simulink model "NGradosLibertadRetoSSControl"  (R2022a)
settings: Solver=VariableStepAuto  StartTime=0.0  StopTime=1000  RelTol=1e-3
undefined symbols (not defined in the file): b, G1, G2, G3, k, L1, L2, L3, m, mbkd_1, mbkd_2, mbkd_3, r_theta_1, r_theta_2, r_theta_3, z_0_1, z_0_2, z_0_3
settings Model: Creator=aafo_  LastModifiedBy=aafo_

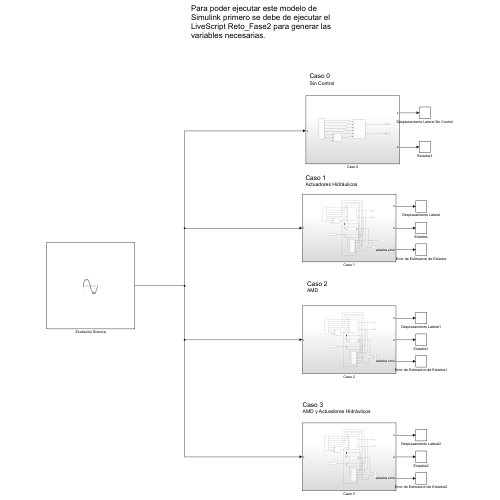
[thumbnail: Simulink's stored preview of the top-level diagram]
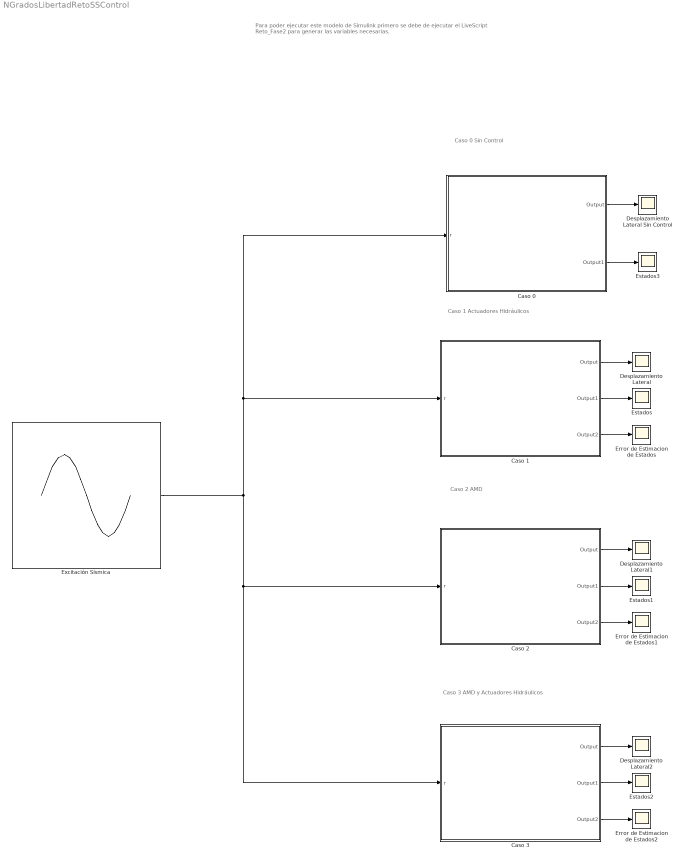
== system NGradosLibertadRetoSSControl ==
  note: Para poder ejecutar este modelo de Simulink primero se debe de ejecutar el LiveScript Reto_Fase2 para generar las variables necesarias.
  note: Caso 1
      | Actuadores Hidráulicos
  note: Caso 2
      | AMD
  note: Caso 3
      | AMD y Actuadores Hidráulicos
  note: Caso 0
      | Sin Control
  Caso 0 : Subsystem
  Caso 1 : Subsystem
  Caso 2 : Subsystem
  Caso 3 : Subsystem
  Desplazamiento Lateral : Scope
  Desplazamiento Lateral Sin Control : Scope
  Desplazamiento Lateral1 : Scope
  Desplazamiento Lateral2 : Scope
  Error de Estimacion de Estados : Scope
  Error de Estimacion de Estados1 : Scope
  Error de Estimacion de Estados2 : Scope
  Estados{,1..3} (4 alike) : Scope
  Excitación Sísmica : Sin  Frequency=14.6165  SampleTime=0
  wires:
  Caso 1/1(Output) -> Desplazamiento Lateral/1
  Caso 1/2(Output1) -> Estados/1
  Caso 1/3(Output2) -> Error de Estimacion de Estados/1
  Caso 2/1(Output) -> Desplazamiento Lateral1/1
  Caso 2/3(Output2) -> Error de Estimacion de Estados1/1
  Caso 2/2(Output1) -> Estados1/1
  Caso 3/2(Output1) -> Estados2/1
  Caso 3/3(Output2) -> Error de Estimacion de Estados2/1
  Caso 3/1(Output) -> Desplazamiento Lateral2/1
  Excitación Sísmica/1 -> Caso 0/1(r), Caso 1/1(r), Caso 3/1(r), Caso 2/1(r)
  Caso 0/2(Output1) -> Estados3/1
  Caso 0/1(Output) -> Desplazamiento Lateral Sin Control/1

== system NGradosLibertadRetoSSControl/Caso 0 ==
  note: Perturbación
  r : Inport
  Parámetros del Sistema : Subsystem
  Perturbacion Matricial : MATLAB Function  TreatAsAtomicUnit=on
  Sistema En Espacio de Estados : Subsystem
  Output : Outport
  Output1 : Outport  Port=2
  wires:
  Perturbacion Matricial/1(out) -> Sistema En Espacio de Estados/6(Perturbación)  "rm"
  Sistema En Espacio de Estados/2(Output6) -> Output1/1  "z"
  Sistema En Espacio de Estados/1(Output5) -> Output/1  "x"
  Parámetros del Sistema/5(Bu) -> Sistema En Espacio de Estados/5(Input4)
  Parámetros del Sistema/3(C) -> Sistema En Espacio de Estados/3(Input2)
  Parámetros del Sistema/1(A) -> Sistema En Espacio de Estados/1(Input)
  Parámetros del Sistema/2(Br) -> Sistema En Espacio de Estados/2(Input1)
  Parámetros del Sistema/7(Output1) -> Perturbacion Matricial/2(m)
  Parámetros del Sistema/4(D) -> Sistema En Espacio de Estados/4(Input3)
  Parámetros del Sistema/6(Output) -> Perturbacion Matricial/1(mbkd)
  r/1 -> Perturbacion Matricial/3(r)

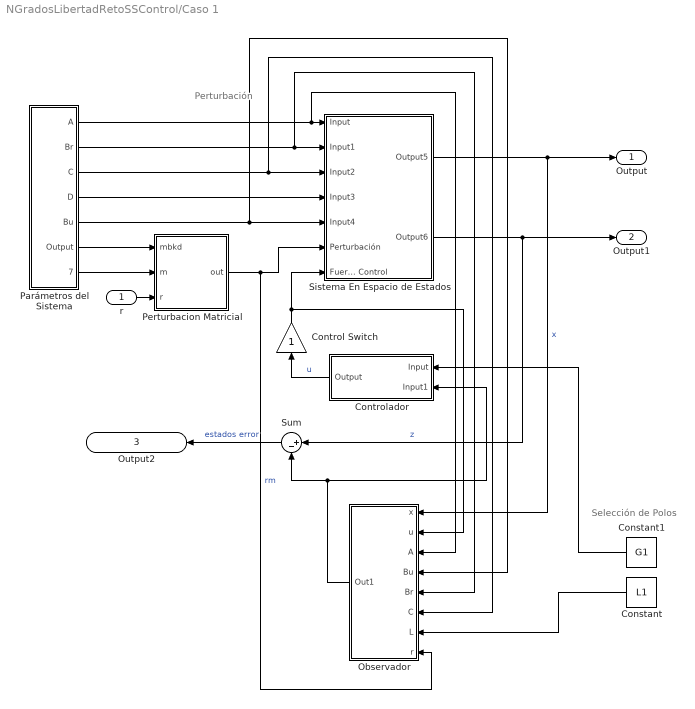
== system NGradosLibertadRetoSSControl/Caso 1 ==
  note: Selección de Polos
  note: Perturbación
  r : Inport
  Constant : Constant  Value=L1
  Constant1 : Constant  Value=G1
  Control Switch : Gain
  Controlador : Subsystem
  Observador : Subsystem
  Parámetros del Sistema : Subsystem
  Perturbacion Matricial : MATLAB Function  TreatAsAtomicUnit=on
  Sistema En Espacio de Estados : Subsystem
  Sum : Sum  Inputs=|+-
  Output : Outport
  Output1 : Outport  Port=2
  Output2 : Outport  Port=3
  wires:
  Observador/1(Out1) -> Controlador/2(Input1), Sum/2
  Sum/1 -> Output2/1  "estados error"
  Perturbacion Matricial/1(out) -> Sistema En Espacio de Estados/6(Perturbación), Observador/8(r)  "rm"
  Sistema En Espacio de Estados/2(Output6) -> Output1/1, Sum/1  "z"
  Sistema En Espacio de Estados/1(Output5) -> Output/1, Observador/1(x)  "x"
  Controlador/1(Output) -> Control Switch/1  "u"
  Parámetros del Sistema/5(Bu) -> Sistema En Espacio de Estados/5(Input4), Observador/4(Bu)
  Parámetros del Sistema/3(C) -> Sistema En Espacio de Estados/3(Input2), Observador/6(C)
  Constant1/1 -> Controlador/1(Input)
  Parámetros del Sistema/1(A) -> Observador/3(A), Sistema En Espacio de Estados/1(Input)
  Parámetros del Sistema/2(Br) -> Sistema En Espacio de Estados/2(Input1), Observador/5(Br)
  Constant/1 -> Observador/7(L)
  Parámetros del Sistema/7(Output1) -> Perturbacion Matricial/2(m)
  Parámetros del Sistema/4(D) -> Sistema En Espacio de Estados/4(Input3)
  Parámetros del Sistema/6(Output) -> Perturbacion Matricial/1(mbkd)
  r/1 -> Perturbacion Matricial/3(r)
  Control Switch/1 -> Sistema En Espacio de Estados/7(Fuerza De Control), Observador/2(u)

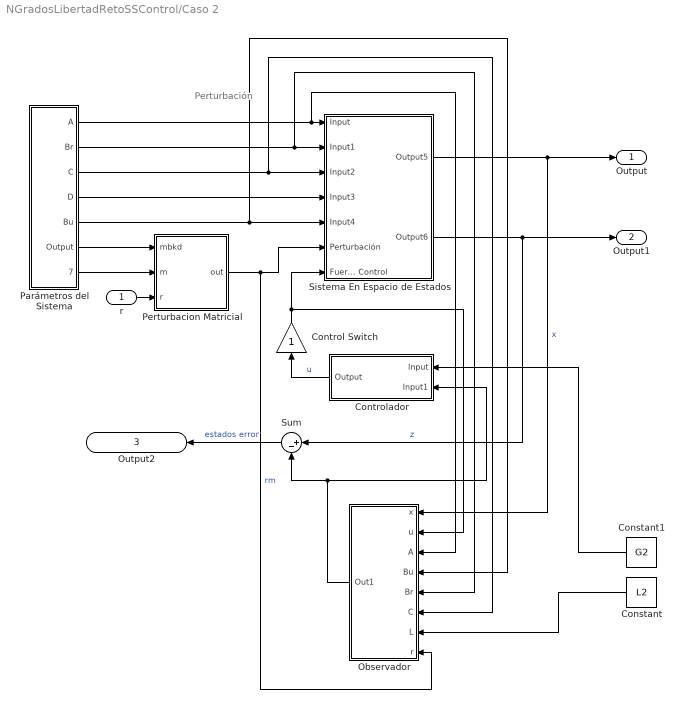
== system NGradosLibertadRetoSSControl/Caso 2 ==
  note: Perturbación
  r : Inport
  Constant : Constant  Value=L2
  Constant1 : Constant  Value=G2
  Control Switch : Gain
  Controlador : Subsystem
  Observador : Subsystem
  Parámetros del Sistema : Subsystem
  Perturbacion Matricial : MATLAB Function  TreatAsAtomicUnit=on
  Sistema En Espacio de Estados : Subsystem
  Sum : Sum  Inputs=|+-
  Output : Outport
  Output1 : Outport  Port=2
  Output2 : Outport  Port=3
  wires:
  Observador/1(Out1) -> Controlador/2(Input1), Sum/2
  Sum/1 -> Output2/1  "estados error"
  Perturbacion Matricial/1(out) -> Sistema En Espacio de Estados/6(Perturbación), Observador/8(r)  "rm"
  Sistema En Espacio de Estados/2(Output6) -> Output1/1, Sum/1  "z"
  Sistema En Espacio de Estados/1(Output5) -> Output/1, Observador/1(x)  "x"
  Controlador/1(Output) -> Control Switch/1  "u"
  Parámetros del Sistema/5(Bu) -> Sistema En Espacio de Estados/5(Input4), Observador/4(Bu)
  Parámetros del Sistema/3(C) -> Sistema En Espacio de Estados/3(Input2), Observador/6(C)
  Constant1/1 -> Controlador/1(Input)
  Parámetros del Sistema/1(A) -> Observador/3(A), Sistema En Espacio de Estados/1(Input)
  Parámetros del Sistema/2(Br) -> Sistema En Espacio de Estados/2(Input1), Observador/5(Br)
  Constant/1 -> Observador/7(L)
  Parámetros del Sistema/7(Output1) -> Perturbacion Matricial/2(m)
  Parámetros del Sistema/4(D) -> Sistema En Espacio de Estados/4(Input3)
  Parámetros del Sistema/6(Output) -> Perturbacion Matricial/1(mbkd)
  r/1 -> Perturbacion Matricial/3(r)
  Control Switch/1 -> Sistema En Espacio de Estados/7(Fuerza De Control), Observador/2(u)

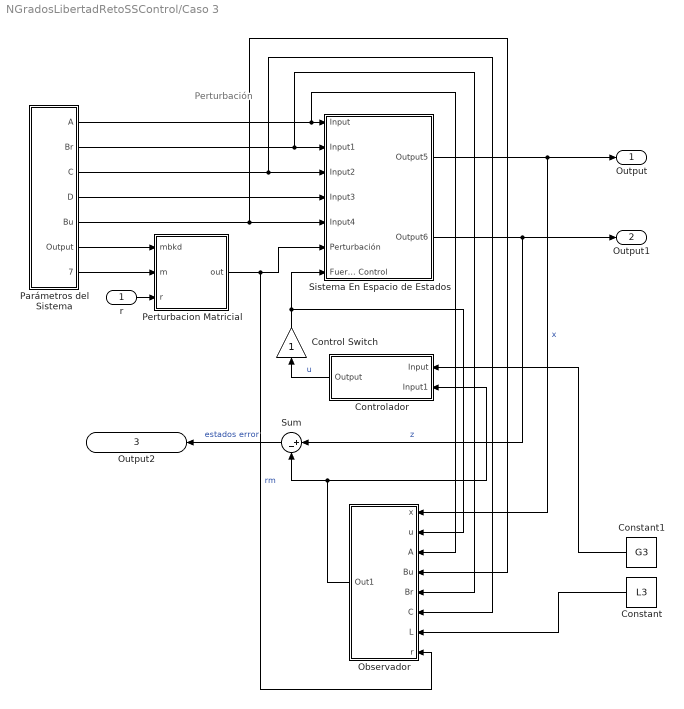
== system NGradosLibertadRetoSSControl/Caso 3 ==
  note: Perturbación
  r : Inport
  Constant : Constant  Value=L3
  Constant1 : Constant  Value=G3
  Control Switch : Gain
  Controlador : Subsystem
  Observador : Subsystem
  Parámetros del Sistema : Subsystem
  Perturbacion Matricial : MATLAB Function  TreatAsAtomicUnit=on
  Sistema En Espacio de Estados : Subsystem
  Sum : Sum  Inputs=|+-
  Output : Outport
  Output1 : Outport  Port=2
  Output2 : Outport  Port=3
  wires:
  Observador/1(Out1) -> Controlador/2(Input1), Sum/2
  Sum/1 -> Output2/1  "estados error"
  Perturbacion Matricial/1(out) -> Sistema En Espacio de Estados/6(Perturbación), Observador/8(r)  "rm"
  Sistema En Espacio de Estados/2(Output6) -> Output1/1, Sum/1  "z"
  Sistema En Espacio de Estados/1(Output5) -> Output/1, Observador/1(x)  "x"
  Controlador/1(Output) -> Control Switch/1  "u"
  Parámetros del Sistema/5(Bu) -> Sistema En Espacio de Estados/5(Input4), Observador/4(Bu)
  Parámetros del Sistema/3(C) -> Sistema En Espacio de Estados/3(Input2), Observador/6(C)
  Constant1/1 -> Controlador/1(Input)
  Parámetros del Sistema/1(A) -> Observador/3(A), Sistema En Espacio de Estados/1(Input)
  Parámetros del Sistema/2(Br) -> Sistema En Espacio de Estados/2(Input1), Observador/5(Br)
  Constant/1 -> Observador/7(L)
  Parámetros del Sistema/7(Output1) -> Perturbacion Matricial/2(m)
  Parámetros del Sistema/4(D) -> Sistema En Espacio de Estados/4(Input3)
  Parámetros del Sistema/6(Output) -> Perturbacion Matricial/1(mbkd)
  r/1 -> Perturbacion Matricial/3(r)
  Control Switch/1 -> Sistema En Espacio de Estados/7(Fuerza De Control), Observador/2(u)

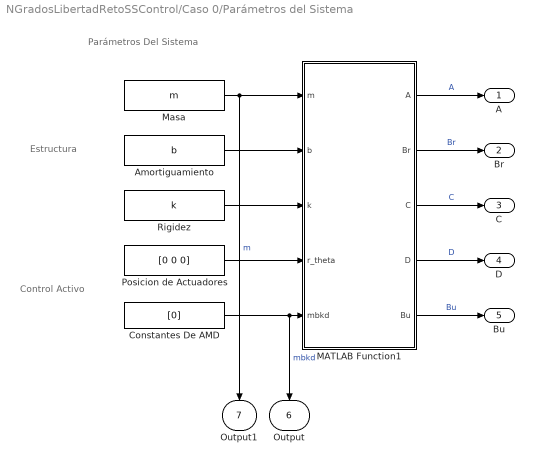
== system NGradosLibertadRetoSSControl/Caso 0/Parámetros del Sistema ==
  note: Control Activo
  note: Estructura
  note: Parámetros Del Sistema
  Amortiguamiento : Constant  Value=b
  Constantes De AMD : Constant  Value=[0]
  MATLAB Function1 : MATLAB Function  TreatAsAtomicUnit=on
  Masa : Constant  Value=m
  Posicion de Actuadores : Constant  Value=[0 0 0]
  Rigidez : Constant  Value=k
  A : Outport
  Br : Outport  Port=2
  C : Outport  Port=3
  D : Outport  Port=4
  Bu : Outport  Port=5
  Output : Outport  Port=6
  Output1 : Outport  Port=7
  wires:
  Masa/1 -> MATLAB Function1/1(m), Output1/1  "m"
  Constantes De AMD/1 -> MATLAB Function1/5(mbkd), Output/1  "mbkd"
  MATLAB Function1/1(A) -> A/1  "A"
  Amortiguamiento/1 -> MATLAB Function1/2(b)
  Rigidez/1 -> MATLAB Function1/3(k)
  Posicion de Actuadores/1 -> MATLAB Function1/4(r_theta)
  MATLAB Function1/2(Br) -> Br/1  "Br"
  MATLAB Function1/3(C) -> C/1  "C"
  MATLAB Function1/4(D) -> D/1  "D"
  MATLAB Function1/5(Bu) -> Bu/1  "Bu"

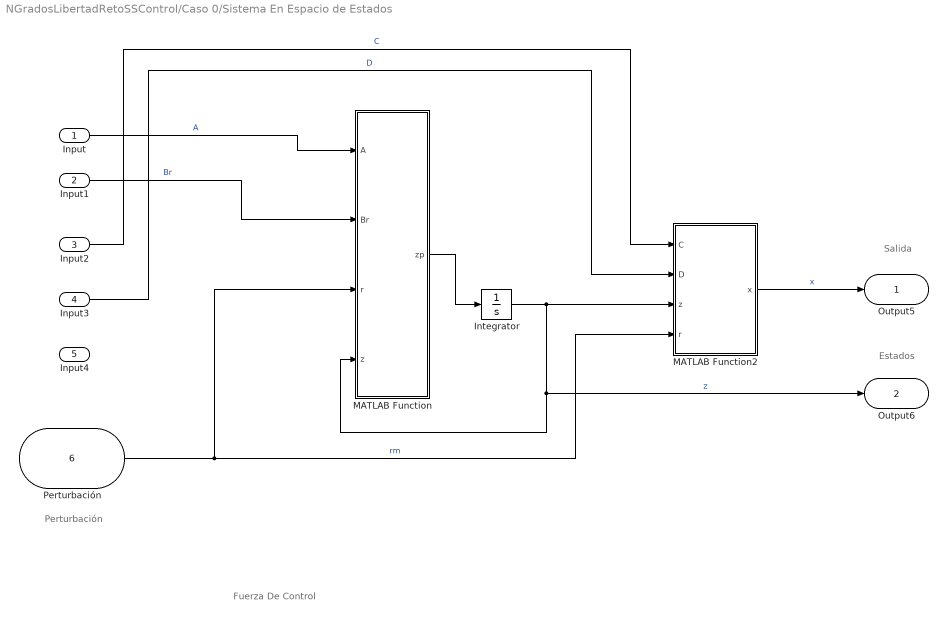
== system NGradosLibertadRetoSSControl/Caso 0/Sistema En Espacio de Estados ==
  note: Estados
  note: Fuerza De Control
  note: Perturbación
  note: Salida
  Input : Inport
  Input1 : Inport  Port=2
  Input2 : Inport  Port=3
  Input3 : Inport  Port=4
  Input4 : Inport  Port=5
  Perturbación : Inport  Port=6
  Integrator : Integrator  InitialCondition=z_0_1
  MATLAB Function : MATLAB Function  TreatAsAtomicUnit=on
  MATLAB Function2 : MATLAB Function  TreatAsAtomicUnit=on
  Output5 : Outport
  Output6 : Outport  Port=2
  wires:
  Integrator/1 -> MATLAB Function/4(z), Output6/1, MATLAB Function2/3(z)  "z"
  Input3/1 -> MATLAB Function2/2(D)  "D"
  Input1/1 -> MATLAB Function/2(Br)  "Br"
  Input/1 -> MATLAB Function/1(A)  "A"
  MATLAB Function/1(zp) -> Integrator/1
  Input2/1 -> MATLAB Function2/1(C)  "C"
  Perturbación/1 -> MATLAB Function2/4(r), MATLAB Function/3(r)  "rm"
  MATLAB Function2/1(x) -> Output5/1  "x"

== system NGradosLibertadRetoSSControl/Caso 1/Controlador ==
  Input : Inport
  Input1 : Inport  Port=2
  Gain : Gain  Gain=-1
  Matrix Multiply : Product  Multiplication=Matrix(*)
  Output : Outport
  wires:
  Input/1 -> Matrix Multiply/1  "G"
  Matrix Multiply/1 -> Gain/1
  Input1/1 -> Matrix Multiply/2  "z"
  Gain/1 -> Output/1  "u"

== system NGradosLibertadRetoSSControl/Caso 1/Observador ==
  x : Inport
  u : Inport  Port=2
  A : Inport  Port=3
  Bu : Inport  Port=4
  Br : Inport  Port=5
  C : Inport  Port=6
  L : Inport  Port=7
  r : Inport  Port=8
  Integrator : Integrator  InitialCondition=z_0_1
  MATLAB Function : MATLAB Function  TreatAsAtomicUnit=on
  Out1 : Outport
  wires:
  Bu/1 -> MATLAB Function/2(Bu)
  MATLAB Function/1(zp_est) -> Integrator/1  "zpest"
  Integrator/1 -> MATLAB Function/9(zest), Out1/1  "zest"
  L/1 -> MATLAB Function/5(L)
  A/1 -> MATLAB Function/1(A)
  Br/1 -> MATLAB Function/3(Br)
  C/1 -> MATLAB Function/4(C)
  r/1 -> MATLAB Function/7(r)
  u/1 -> MATLAB Function/6(u)
  x/1 -> MATLAB Function/8(x)

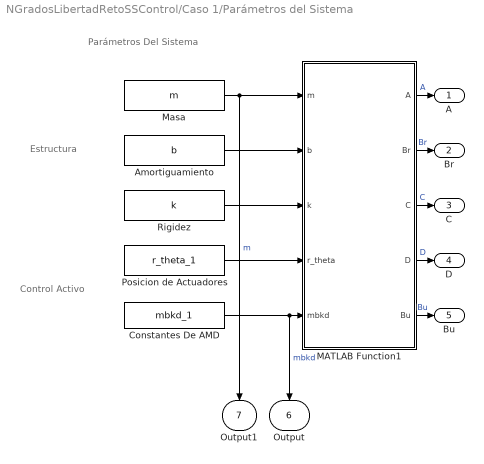
== system NGradosLibertadRetoSSControl/Caso 1/Parámetros del Sistema ==
  note: Control Activo
  note: Estructura
  note: Parámetros Del Sistema
  Amortiguamiento : Constant  Value=b
  Constantes De AMD : Constant  Value=mbkd_1
  MATLAB Function1 : MATLAB Function  TreatAsAtomicUnit=on
  Masa : Constant  Value=m
  Posicion de Actuadores : Constant  Value=r_theta_1
  Rigidez : Constant  Value=k
  A : Outport
  Br : Outport  Port=2
  C : Outport  Port=3
  D : Outport  Port=4
  Bu : Outport  Port=5
  Output : Outport  Port=6
  Output1 : Outport  Port=7
  wires:
  Masa/1 -> MATLAB Function1/1(m), Output1/1  "m"
  Constantes De AMD/1 -> MATLAB Function1/5(mbkd), Output/1  "mbkd"
  MATLAB Function1/1(A) -> A/1  "A"
  Amortiguamiento/1 -> MATLAB Function1/2(b)
  Rigidez/1 -> MATLAB Function1/3(k)
  Posicion de Actuadores/1 -> MATLAB Function1/4(r_theta)
  MATLAB Function1/2(Br) -> Br/1  "Br"
  MATLAB Function1/3(C) -> C/1  "C"
  MATLAB Function1/4(D) -> D/1  "D"
  MATLAB Function1/5(Bu) -> Bu/1  "Bu"

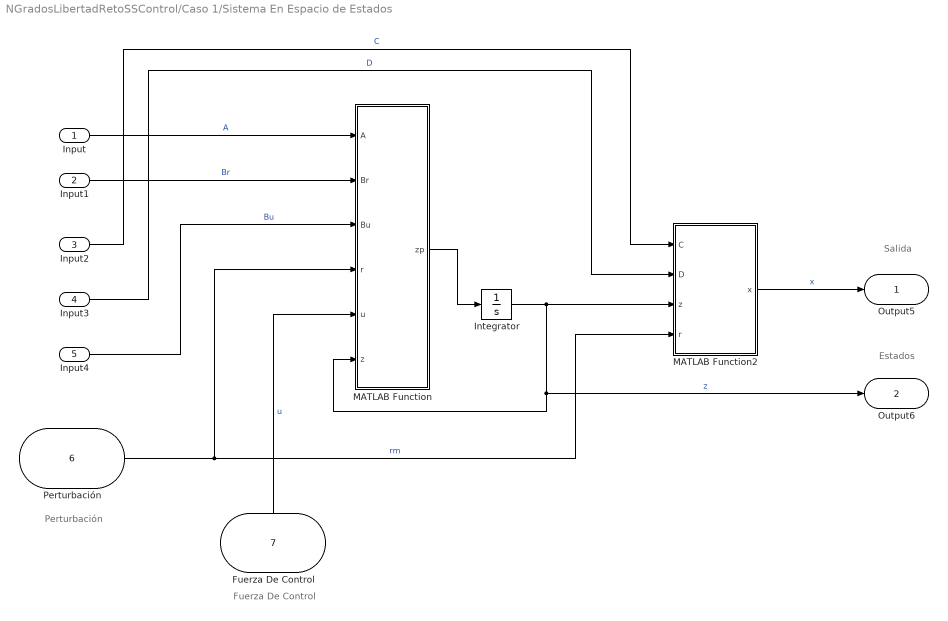
== system NGradosLibertadRetoSSControl/Caso 1/Sistema En Espacio de Estados ==
  note: Estados
  note: Fuerza De Control
  note: Perturbación
  note: Salida
  Input : Inport
  Input1 : Inport  Port=2
  Input2 : Inport  Port=3
  Input3 : Inport  Port=4
  Input4 : Inport  Port=5
  Perturbación : Inport  Port=6
  Fuerza De Control : Inport  Port=7
  Integrator : Integrator  InitialCondition=z_0_1
  MATLAB Function : MATLAB Function  TreatAsAtomicUnit=on
  MATLAB Function2 : MATLAB Function  TreatAsAtomicUnit=on
  Output5 : Outport
  Output6 : Outport  Port=2
  wires:
  Integrator/1 -> MATLAB Function/6(z), Output6/1, MATLAB Function2/3(z)  "z"
  Input3/1 -> MATLAB Function2/2(D)  "D"
  Input1/1 -> MATLAB Function/2(Br)  "Br"
  Input/1 -> MATLAB Function/1(A)  "A"
  MATLAB Function/1(zp) -> Integrator/1
  Input2/1 -> MATLAB Function2/1(C)  "C"
  Perturbación/1 -> MATLAB Function2/4(r), MATLAB Function/4(r)  "rm"
  MATLAB Function2/1(x) -> Output5/1  "x"
  Input4/1 -> MATLAB Function/3(Bu)  "Bu"
  Fuerza De Control/1 -> MATLAB Function/5(u)  "u"

== system NGradosLibertadRetoSSControl/Caso 2/Controlador ==
  Input : Inport
  Input1 : Inport  Port=2
  Gain : Gain  Gain=-1
  Matrix Multiply : Product  Multiplication=Matrix(*)
  Output : Outport
  wires:
  Input/1 -> Matrix Multiply/1  "G"
  Matrix Multiply/1 -> Gain/1
  Input1/1 -> Matrix Multiply/2  "z"
  Gain/1 -> Output/1  "u"

== system NGradosLibertadRetoSSControl/Caso 2/Observador ==
  x : Inport
  u : Inport  Port=2
  A : Inport  Port=3
  Bu : Inport  Port=4
  Br : Inport  Port=5
  C : Inport  Port=6
  L : Inport  Port=7
  r : Inport  Port=8
  Integrator : Integrator  InitialCondition=z_0_2
  MATLAB Function : MATLAB Function  TreatAsAtomicUnit=on
  Out1 : Outport
  wires:
  Bu/1 -> MATLAB Function/2(Bu)
  MATLAB Function/1(zp_est) -> Integrator/1  "zpest"
  Integrator/1 -> MATLAB Function/9(zest), Out1/1  "zest"
  L/1 -> MATLAB Function/5(L)
  A/1 -> MATLAB Function/1(A)
  Br/1 -> MATLAB Function/3(Br)
  C/1 -> MATLAB Function/4(C)
  r/1 -> MATLAB Function/7(r)
  u/1 -> MATLAB Function/6(u)
  x/1 -> MATLAB Function/8(x)

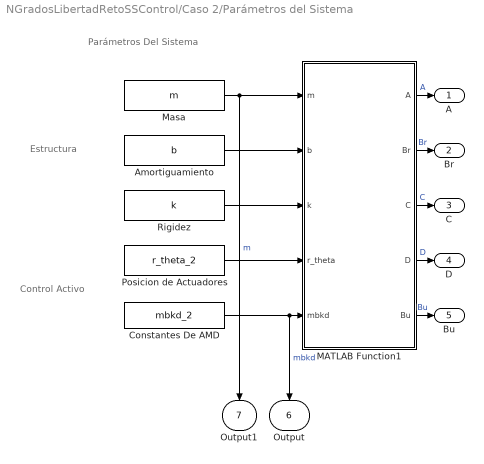
== system NGradosLibertadRetoSSControl/Caso 2/Parámetros del Sistema ==
  note: Control Activo
  note: Estructura
  note: Parámetros Del Sistema
  Amortiguamiento : Constant  Value=b
  Constantes De AMD : Constant  Value=mbkd_2
  MATLAB Function1 : MATLAB Function  TreatAsAtomicUnit=on
  Masa : Constant  Value=m
  Posicion de Actuadores : Constant  Value=r_theta_2
  Rigidez : Constant  Value=k
  A : Outport
  Br : Outport  Port=2
  C : Outport  Port=3
  D : Outport  Port=4
  Bu : Outport  Port=5
  Output : Outport  Port=6
  Output1 : Outport  Port=7
  wires:
  Masa/1 -> MATLAB Function1/1(m), Output1/1  "m"
  Constantes De AMD/1 -> MATLAB Function1/5(mbkd), Output/1  "mbkd"
  MATLAB Function1/1(A) -> A/1  "A"
  Amortiguamiento/1 -> MATLAB Function1/2(b)
  Rigidez/1 -> MATLAB Function1/3(k)
  Posicion de Actuadores/1 -> MATLAB Function1/4(r_theta)
  MATLAB Function1/2(Br) -> Br/1  "Br"
  MATLAB Function1/3(C) -> C/1  "C"
  MATLAB Function1/4(D) -> D/1  "D"
  MATLAB Function1/5(Bu) -> Bu/1  "Bu"

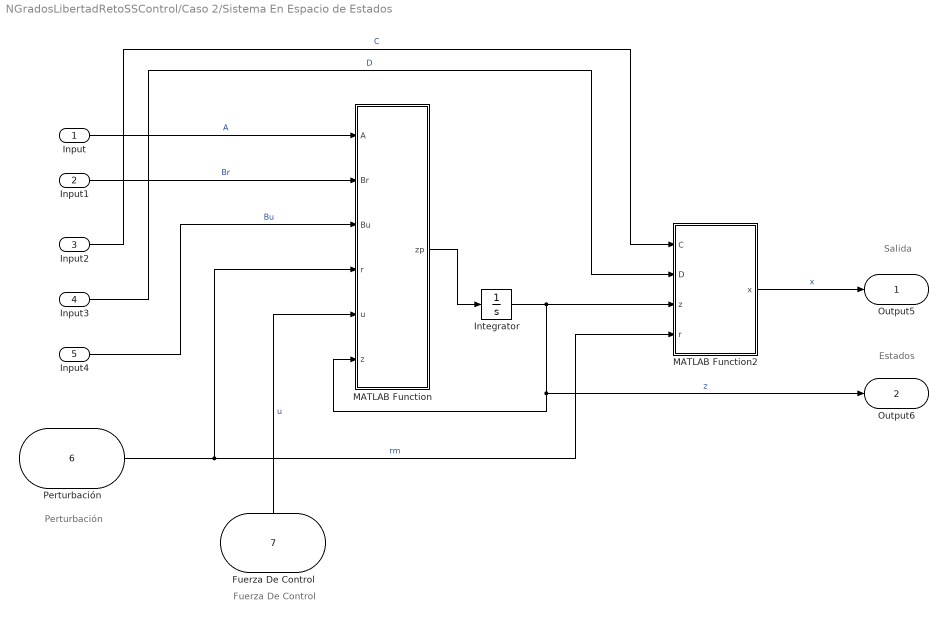
== system NGradosLibertadRetoSSControl/Caso 2/Sistema En Espacio de Estados ==
  note: Estados
  note: Fuerza De Control
  note: Perturbación
  note: Salida
  Input : Inport
  Input1 : Inport  Port=2
  Input2 : Inport  Port=3
  Input3 : Inport  Port=4
  Input4 : Inport  Port=5
  Perturbación : Inport  Port=6
  Fuerza De Control : Inport  Port=7
  Integrator : Integrator  InitialCondition=z_0_2
  MATLAB Function : MATLAB Function  TreatAsAtomicUnit=on
  MATLAB Function2 : MATLAB Function  TreatAsAtomicUnit=on
  Output5 : Outport
  Output6 : Outport  Port=2
  wires:
  Integrator/1 -> MATLAB Function/6(z), Output6/1, MATLAB Function2/3(z)  "z"
  Input3/1 -> MATLAB Function2/2(D)  "D"
  Input1/1 -> MATLAB Function/2(Br)  "Br"
  Input/1 -> MATLAB Function/1(A)  "A"
  MATLAB Function/1(zp) -> Integrator/1
  Input2/1 -> MATLAB Function2/1(C)  "C"
  Perturbación/1 -> MATLAB Function2/4(r), MATLAB Function/4(r)  "rm"
  MATLAB Function2/1(x) -> Output5/1  "x"
  Input4/1 -> MATLAB Function/3(Bu)  "Bu"
  Fuerza De Control/1 -> MATLAB Function/5(u)  "u"

== system NGradosLibertadRetoSSControl/Caso 3/Controlador ==
  Input : Inport
  Input1 : Inport  Port=2
  Gain : Gain  Gain=-1
  Matrix Multiply : Product  Multiplication=Matrix(*)
  Output : Outport
  wires:
  Input/1 -> Matrix Multiply/1  "G"
  Matrix Multiply/1 -> Gain/1
  Input1/1 -> Matrix Multiply/2  "z"
  Gain/1 -> Output/1  "u"

== system NGradosLibertadRetoSSControl/Caso 3/Observador ==
  x : Inport
  u : Inport  Port=2
  A : Inport  Port=3
  Bu : Inport  Port=4
  Br : Inport  Port=5
  C : Inport  Port=6
  L : Inport  Port=7
  r : Inport  Port=8
  Integrator : Integrator  InitialCondition=z_0_3
  MATLAB Function : MATLAB Function  TreatAsAtomicUnit=on
  Out1 : Outport
  wires:
  Bu/1 -> MATLAB Function/2(Bu)
  MATLAB Function/1(zp_est) -> Integrator/1  "zpest"
  Integrator/1 -> MATLAB Function/9(zest), Out1/1  "zest"
  L/1 -> MATLAB Function/5(L)
  A/1 -> MATLAB Function/1(A)
  Br/1 -> MATLAB Function/3(Br)
  C/1 -> MATLAB Function/4(C)
  r/1 -> MATLAB Function/7(r)
  u/1 -> MATLAB Function/6(u)
  x/1 -> MATLAB Function/8(x)

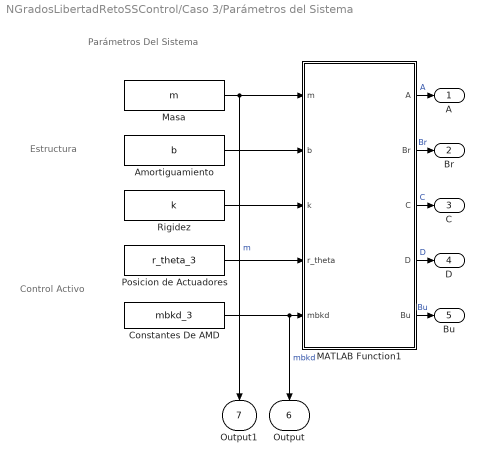
== system NGradosLibertadRetoSSControl/Caso 3/Parámetros del Sistema ==
  note: Control Activo
  note: Estructura
  note: Parámetros Del Sistema
  Amortiguamiento : Constant  Value=b
  Constantes De AMD : Constant  Value=mbkd_3
  MATLAB Function1 : MATLAB Function  TreatAsAtomicUnit=on
  Masa : Constant  Value=m
  Posicion de Actuadores : Constant  Value=r_theta_3
  Rigidez : Constant  Value=k
  A : Outport
  Br : Outport  Port=2
  C : Outport  Port=3
  D : Outport  Port=4
  Bu : Outport  Port=5
  Output : Outport  Port=6
  Output1 : Outport  Port=7
  wires:
  Masa/1 -> MATLAB Function1/1(m), Output1/1  "m"
  Constantes De AMD/1 -> MATLAB Function1/5(mbkd), Output/1  "mbkd"
  MATLAB Function1/1(A) -> A/1  "A"
  Amortiguamiento/1 -> MATLAB Function1/2(b)
  Rigidez/1 -> MATLAB Function1/3(k)
  Posicion de Actuadores/1 -> MATLAB Function1/4(r_theta)
  MATLAB Function1/2(Br) -> Br/1  "Br"
  MATLAB Function1/3(C) -> C/1  "C"
  MATLAB Function1/4(D) -> D/1  "D"
  MATLAB Function1/5(Bu) -> Bu/1  "Bu"

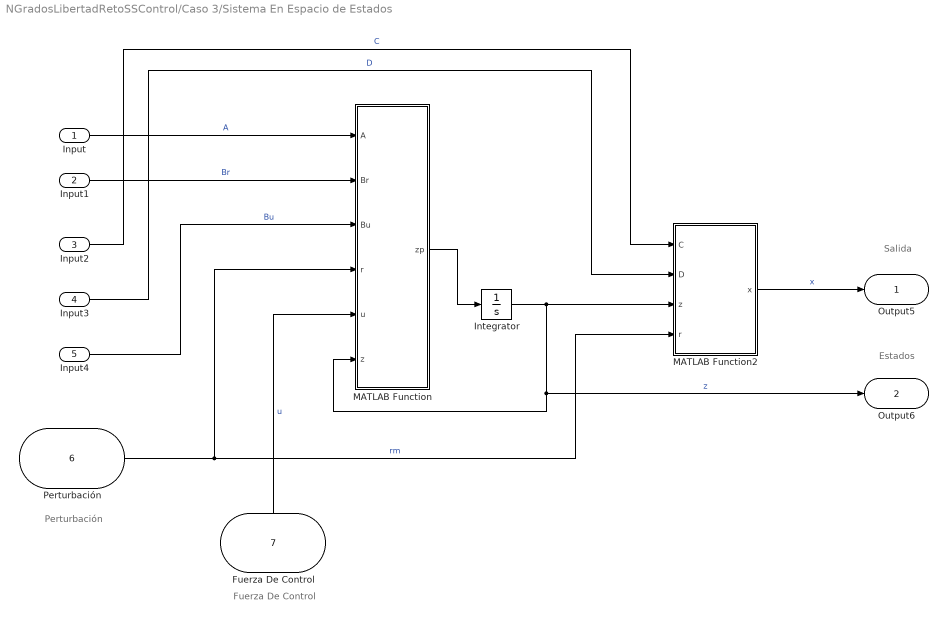
== system NGradosLibertadRetoSSControl/Caso 3/Sistema En Espacio de Estados ==
  note: Estados
  note: Fuerza De Control
  note: Perturbación
  note: Salida
  Input : Inport
  Input1 : Inport  Port=2
  Input2 : Inport  Port=3
  Input3 : Inport  Port=4
  Input4 : Inport  Port=5
  Perturbación : Inport  Port=6
  Fuerza De Control : Inport  Port=7
  Integrator : Integrator  InitialCondition=z_0_3
  MATLAB Function : MATLAB Function  TreatAsAtomicUnit=on
  MATLAB Function2 : MATLAB Function  TreatAsAtomicUnit=on
  Output5 : Outport
  Output6 : Outport  Port=2
  wires:
  Integrator/1 -> MATLAB Function/6(z), Output6/1, MATLAB Function2/3(z)  "z"
  Input3/1 -> MATLAB Function2/2(D)  "D"
  Input1/1 -> MATLAB Function/2(Br)  "Br"
  Input/1 -> MATLAB Function/1(A)  "A"
  MATLAB Function/1(zp) -> Integrator/1
  Input2/1 -> MATLAB Function2/1(C)  "C"
  Perturbación/1 -> MATLAB Function2/4(r), MATLAB Function/4(r)  "rm"
  MATLAB Function2/1(x) -> Output5/1  "x"
  Input4/1 -> MATLAB Function/3(Bu)  "Bu"
  Fuerza De Control/1 -> MATLAB Function/5(u)  "u"

== matlab function NGradosLibertadRetoSSControl/Caso 2/Perturbacion Matricial ==
  data: mbkd input; m input; r input; out output
function out = rMatrix(mbkd, m,r)
n = length(m);
if length(mbkd) == 3

    out = r.*ones(n+1,1);
else
    out = r.*ones(n,1);
end

== matlab function NGradosLibertadRetoSSControl/Caso 2/Sistema En Espacio de Estados/MATLAB Function ==
  data: A input; Br input; Bu input; r input; u input; z input; zp output
function zp = StatesModel(A , Br, Bu, r, u, z)

zp = A*z+Br*r+ Bu*u;

== matlab function NGradosLibertadRetoSSControl/Caso 2/Sistema En Espacio de Estados/MATLAB Function2 ==
  data: C input; D input; z input; x output; r input
function x = StatesToX(C, D, z, r)

x = C*z+ D*r;

== matlab function NGradosLibertadRetoSSControl/Caso 3/Observador/MATLAB Function ==
  data: A input; Bu input; Br input; C input; L input; u input; zp_est output; r input; x input; zest input
function zp_est = fcn(A, Bu, Br, C, L, u, r, x, zest)

xerr = x-C*zest;
zp_est = A*zest + Bu*u + Br*r + L*xerr;

== matlab function NGradosLibertadRetoSSControl/Caso 3/Parámetros del Sistema/MATLAB Function1 ==
  data: m input; A output; b input; k input; r_theta input; Br output; C output; D output; Bu output; mbkd input
function [A, Br, C, D, Bu] = StatesModelMatrix(m, b, k, r_theta, mbkd)
if length(mbkd) == 3
%% AMD
    md = mbkd(1); bd = mbkd(2); kd = mbkd(3);

    M = MM_AMD(MM(m),md);
    
    B_ = BK_AMD(BK(b),bd);
    
    K = BK_AMD(BK(k),kd);
    
    delta = -1*[m' md]';
    
    nn = size(M, 1);
    
    gamma = gamma_AMD(gamma_bar(length(m))*MM(r_theta));
    
    A = [zeros(nn) eye(nn); -inv(M)*K -inv(M)*B_];
    
    Br = [zeros(nn);MM(inv(M)*delta)];
    
    Bu = [zeros(nn); inv(M)*gamma];
    
    C = [eye(nn) zeros(nn)];
    
    D = zeros(nn);

%% Sin AMD
else

    M = MM(m);
    
    B_ = BK(b);
    
    K = BK(k);
    
    delta = -1*m;
    
    nn = size(M, 1);
    
    gamma = gamma_bar(length(m))*MM(r_theta);
    
    A = [zeros(nn) eye(nn); -inv(M)*K -inv(M)*B_];
    
    Br = [zeros(nn);MM(inv(M)*delta)];
    
    Bu = [zeros(nn); inv(M)*gamma];
    
    C = [eye(nn) zeros(nn)];
    
    D = zeros(nn);

end
%% Funciones de Matrices
function matrix = BK(el)

n = length(el);
matrix = zeros(n);

for i = 1:n
    for j = 1:n
        if j == i+1
            matrix(i,j) = -el(i+1);
        elseif j == i-1
            matrix(i,j) = -el(i);
        elseif i==j
            if  i == n && j == n
                matrix(i,j) = el(n);
            else
                matrix(i,j) = el(i)+el(i+1);
            end
        else
            matrix(i,j) = 0;
        end
    end
end
end

function matrix = MM(el)

n = length(el);
matrix = zeros(n);

for i = 1:n
    matrix(i,i) = el(i);

end
end

function matrix = BK_AMD(mat, el)
n = size(mat, 1);
matrix = [mat zeros(n,1); zeros(1,n-1) -el el];
end

function matrix = gamma_bar(n)

matrix = zeros(n);

for i = 1:n
   if i ~= n
        matrix(i, i) = -1;
        matrix(i, i+1) = 1; 
   else 
       matrix(i,i) = -1;
   end
end
end

function matrix = gamma_AMD(mat)
n = size(mat, 1);
matrix = [mat [zeros(n-1,1);-1];zeros(1,n) 1];

end

function matrix = MM_AMD(mat, el)

n = size(mat, 1);

matrix = [mat zeros(n, 1);zeros(1,n) el];

end
end

== matlab function NGradosLibertadRetoSSControl/Caso 3/Perturbacion Matricial ==
  data: mbkd input; m input; r input; out output
function out = rMatrix(mbkd, m,r)
n = length(m);
if length(mbkd) == 3

    out = r.*ones(n+1,1);
else
    out = r.*ones(n,1);
end

== matlab function NGradosLibertadRetoSSControl/Caso 1/Parámetros del Sistema/MATLAB Function1 ==
  data: m input; A output; b input; k input; r_theta input; Br output; C output; D output; Bu output; mbkd input
function [A, Br, C, D, Bu] = StatesModelMatrix(m, b, k, r_theta, mbkd)
if length(mbkd) == 3
%% AMD
    md = mbkd(1); bd = mbkd(2); kd = mbkd(3);

    M = MM_AMD(MM(m),md);
    
    B_ = BK_AMD(BK(b),bd);
    
    K = BK_AMD(BK(k),kd);
    
    delta = -1*[m' md]';
    
    nn = size(M, 1);
    
    gamma = gamma_AMD(gamma_bar(length(m))*MM(r_theta));
    
    A = [zeros(nn) eye(nn); -inv(M)*K -inv(M)*B_];
    
    Br = [zeros(nn);MM(inv(M)*delta)];
    
    Bu = [zeros(nn); inv(M)*gamma];
    
    C = [eye(nn) zeros(nn)];
    
    D = zeros(nn);

%% Sin AMD
else

    M = MM(m);
    
    B_ = BK(b);
    
    K = BK(k);
    
    delta = -1*m;
    
    nn = size(M, 1);
    
    gamma = gamma_bar(length(m))*MM(r_theta);
    
    A = [zeros(nn) eye(nn); -inv(M)*K -inv(M)*B_];
    
    Br = [zeros(nn);MM(inv(M)*delta)];
    
    Bu = [zeros(nn); inv(M)*gamma];
    
    C = [eye(nn) zeros(nn)];
    
    D = zeros(nn);

end
%% Funciones de Matrices
function matrix = BK(el)

n = length(el);
matrix = zeros(n);

for i = 1:n
    for j = 1:n
        if j == i+1
            matrix(i,j) = -el(i+1);
        elseif j == i-1
            matrix(i,j) = -el(i);
        elseif i==j
            if  i == n && j == n
                matrix(i,j) = el(n);
            else
                matrix(i,j) = el(i)+el(i+1);
            end
        else
            matrix(i,j) = 0;
        end
    end
end
end

function matrix = MM(el)

n = length(el);
matrix = zeros(n);

for i = 1:n
    matrix(i,i) = el(i);

end
end

function matrix = BK_AMD(mat, el)
n = size(mat, 1);
matrix = [mat zeros(n,1); zeros(1,n-1) -el el];
end

function matrix = gamma_bar(n)

matrix = zeros(n);

for i = 1:n
   if i ~= n
        matrix(i, i) = -1;
        matrix(i, i+1) = 1; 
   else 
       matrix(i,i) = -1;
   end
end
end

function matrix = gamma_AMD(mat)
n = size(mat, 1);
matrix = [mat [zeros(n-1,1);-1];zeros(1,n) 1];

end

function matrix = MM_AMD(mat, el)

n = size(mat, 1);

matrix = [mat zeros(n, 1);zeros(1,n) el];

end
end

== matlab function NGradosLibertadRetoSSControl/Caso 3/Sistema En Espacio de Estados/MATLAB Function ==
  data: A input; Br input; Bu input; r input; u input; z input; zp output
function zp = StatesModel(A , Br, Bu, r, u, z)

zp = A*z+Br*r+ Bu*u;

== matlab function NGradosLibertadRetoSSControl/Caso 3/Sistema En Espacio de Estados/MATLAB Function2 ==
  data: C input; D input; z input; x output; r input
function x = StatesToX(C, D, z, r)

x = C*z+ D*r;

== matlab function NGradosLibertadRetoSSControl/Caso 0/Parámetros del Sistema/MATLAB Function1 ==
  data: m input; A output; b input; k input; r_theta input; Br output; C output; D output; Bu output; mbkd input
function [A, Br, C, D, Bu] = StatesModelMatrix(m, b, k, r_theta, mbkd)
if length(mbkd) == 3
%% AMD
    md = mbkd(1); bd = mbkd(2); kd = mbkd(3);

    M = MM_AMD(MM(m),md);
    
    B_ = BK_AMD(BK(b),bd);
    
    K = BK_AMD(BK(k),kd);
    
    delta = -1*[m' md]';
    
    nn = size(M, 1);
    
    gamma = gamma_AMD(gamma_bar(length(m))*MM(r_theta));
    
    A = [zeros(nn) eye(nn); -inv(M)*K -inv(M)*B_];
    
    Br = [zeros(nn);MM(inv(M)*delta)];
    
    Bu = [zeros(nn); inv(M)*gamma];
    
    C = [eye(nn) zeros(nn)];
    
    D = zeros(nn);

%% Sin AMD
else

    M = MM(m);
    
    B_ = BK(b);
    
    K = BK(k);
    
    delta = -1*m;
    
    nn = size(M, 1);
    
    gamma = gamma_bar(length(m))*MM(r_theta);
    
    A = [zeros(nn) eye(nn); -inv(M)*K -inv(M)*B_];
    
    Br = [zeros(nn);MM(inv(M)*delta)];
    
    Bu = [zeros(nn); inv(M)*gamma];
    
    C = [eye(nn) zeros(nn)];
    
    D = zeros(nn);

end
%% Funciones de Matrices
function matrix = BK(el)

n = length(el);
matrix = zeros(n);

for i = 1:n
    for j = 1:n
        if j == i+1
            matrix(i,j) = -el(i+1);
        elseif j == i-1
            matrix(i,j) = -el(i);
        elseif i==j
            if  i == n && j == n
                matrix(i,j) = el(n);
            else
                matrix(i,j) = el(i)+el(i+1);
            end
        else
            matrix(i,j) = 0;
        end
    end
end
end

function matrix = MM(el)

n = length(el);
matrix = zeros(n);

for i = 1:n
    matrix(i,i) = el(i);

end
end

function matrix = BK_AMD(mat, el)
n = size(mat, 1);
matrix = [mat zeros(n,1); zeros(1,n-1) -el el];
end

function matrix = gamma_bar(n)

matrix = zeros(n);

for i = 1:n
   if i ~= n
        matrix(i, i) = -1;
        matrix(i, i+1) = 1; 
   else 
       matrix(i,i) = -1;
   end
end
end

function matrix = gamma_AMD(mat)
n = size(mat, 1);
matrix = [mat [zeros(n-1,1);-1];zeros(1,n) 1];

end

function matrix = MM_AMD(mat, el)

n = size(mat, 1);

matrix = [mat zeros(n, 1);zeros(1,n) el];

end
end

== matlab function NGradosLibertadRetoSSControl/Caso 0/Perturbacion Matricial ==
  data: mbkd input; m input; r input; out output
function out = rMatrix(mbkd, m,r)
n = length(m);
if length(mbkd) == 3

    out = r.*ones(n+1,1);
else
    out = r.*ones(n,1);
end

== matlab function NGradosLibertadRetoSSControl/Caso 0/Sistema En Espacio de Estados/MATLAB Function ==
  data: A input; Br input; r input; z input; zp output
function zp = StatesModel(A , Br, r, z)

zp = A*z+Br*r;

== matlab function NGradosLibertadRetoSSControl/Caso 0/Sistema En Espacio de Estados/MATLAB Function2 ==
  data: C input; D input; z input; x output; r input
function x = StatesToX(C, D, z, r)

x = C*z+ D*r;

== matlab function NGradosLibertadRetoSSControl/Caso 1/Sistema En Espacio de Estados/MATLAB Function ==
  data: A input; Br input; Bu input; r input; u input; z input; zp output
function zp = StatesModel(A , Br, Bu, r, u, z)

zp = A*z+Br*r+ Bu*u;

== matlab function NGradosLibertadRetoSSControl/Caso 1/Perturbacion Matricial ==
  data: mbkd input; m input; r input; out output
function out = rMatrix(mbkd, m,r)
n = length(m);
if length(mbkd) == 3

    out = r.*ones(n+1,1);
else
    out = r.*ones(n,1);
end

== matlab function NGradosLibertadRetoSSControl/Caso 1/Sistema En Espacio de Estados/MATLAB Function2 ==
  data: C input; D input; z input; x output; r input
function x = StatesToX(C, D, z, r)

x = C*z+ D*r;

== matlab function NGradosLibertadRetoSSControl/Caso 1/Observador/MATLAB Function ==
  data: A input; Bu input; Br input; C input; L input; u input; zp_est output; r input; x input; zest input
function zp_est = fcn(A, Bu, Br, C, L, u, r, x, zest)

xerr = x-C*zest;
zp_est = A*zest + Bu*u + Br*r + L*xerr;

== matlab function NGradosLibertadRetoSSControl/Caso 2/Observador/MATLAB Function ==
  data: A input; Bu input; Br input; C input; L input; u input; zp_est output; r input; x input; zest input
function zp_est = fcn(A, Bu, Br, C, L, u, r, x, zest)

xerr = x-C*zest;
zp_est = A*zest + Bu*u + Br*r + L*xerr;

== matlab function NGradosLibertadRetoSSControl/Caso 2/Parámetros del Sistema/MATLAB Function1 ==
  data: m input; A output; b input; k input; r_theta input; Br output; C output; D output; Bu output; mbkd input
function [A, Br, C, D, Bu] = StatesModelMatrix(m, b, k, r_theta, mbkd)
if length(mbkd) == 3
%% AMD
    md = mbkd(1); bd = mbkd(2); kd = mbkd(3);

    M = MM_AMD(MM(m),md);
    
    B_ = BK_AMD(BK(b),bd);
    
    K = BK_AMD(BK(k),kd);
    
    delta = -1*[m' md]';
    
    nn = size(M, 1);
    
    gamma = gamma_AMD(gamma_bar(length(m))*MM(r_theta));
    
    A = [zeros(nn) eye(nn); -inv(M)*K -inv(M)*B_];
    
    Br = [zeros(nn);MM(inv(M)*delta)];
    
    Bu = [zeros(nn); inv(M)*gamma];
    
    C = [eye(nn) zeros(nn)];
    
    D = zeros(nn);

%% Sin AMD
else

    M = MM(m);
    
    B_ = BK(b);
    
    K = BK(k);
    
    delta = -1*m;
    
    nn = size(M, 1);
    
    gamma = gamma_bar(length(m))*MM(r_theta);
    
    A = [zeros(nn) eye(nn); -inv(M)*K -inv(M)*B_];
    
    Br = [zeros(nn);MM(inv(M)*delta)];
    
    Bu = [zeros(nn); inv(M)*gamma];
    
    C = [eye(nn) zeros(nn)];
    
    D = zeros(nn);

end
%% Funciones de Matrices
function matrix = BK(el)

n = length(el);
matrix = zeros(n);

for i = 1:n
    for j = 1:n
        if j == i+1
            matrix(i,j) = -el(i+1);
        elseif j == i-1
            matrix(i,j) = -el(i);
        elseif i==j
            if  i == n && j == n
                matrix(i,j) = el(n);
            else
                matrix(i,j) = el(i)+el(i+1);
            end
        else
            matrix(i,j) = 0;
        end
    end
end
end

function matrix = MM(el)

n = length(el);
matrix = zeros(n);

for i = 1:n
    matrix(i,i) = el(i);

end
end

function matrix = BK_AMD(mat, el)
n = size(mat, 1);
matrix = [mat zeros(n,1); zeros(1,n-1) -el el];
end

function matrix = gamma_bar(n)

matrix = zeros(n);

for i = 1:n
   if i ~= n
        matrix(i, i) = -1;
        matrix(i, i+1) = 1; 
   else 
       matrix(i,i) = -1;
   end
end
end

function matrix = gamma_AMD(mat)
n = size(mat, 1);
matrix = [mat [zeros(n-1,1);-1];zeros(1,n) 1];

end

function matrix = MM_AMD(mat, el)

n = size(mat, 1);

matrix = [mat zeros(n, 1);zeros(1,n) el];

end
end
